simulink model "FOC_IM_1"  (R2021a)
settings: Solver=VariableStepAuto  StartTime=0.0  StopTime=10.0  RelTol=1e-3
values from neighbouring files (symbols this model uses):
  dataType = 'single'    [FOC_IM_1.m]
  inverter = mcb_SetInverterParameters('BoostXL-DRV8305')    [FOC_IM_1.m]
  PI_params = mcb.internal.SetControllerParameters(acim,inverter,PU_System,T_pwm,Ts,Ts_speed,Delays)    [FOC_IM_1.m]
  PU_System = mcb_SetPUSystem(acim,inverter)    [FOC_IM_1.m]
  target = mcb_SetProcessorDetails('F28379D',PWM_frequency)    [FOC_IM_1.m]
  Ts = T_pwm    (= 5e-05)    [FOC_IM_1.m]
  Ts_motor = T_pwm/2    (= 2.5e-05)    [FOC_IM_1.m]
  Ts_simulink = T_pwm/2    (= 2.5e-05)    [FOC_IM_1.m]
  Ts_speed = 30*Ts    (= 0.0015)    [FOC_IM_1.m]
undefined symbols (not defined in the file or in its folder): acim, IIR_filter_speed
libraries: mcbcontrolslib x21, simulink x8, c280xlib x3, mcbpositiondecoderlib x3, c2802xlib x2, autolibim x1, mcbplantlib x1, fuzblock x1
settings Model: Creator=ACER  LastModifiedBy=ACER

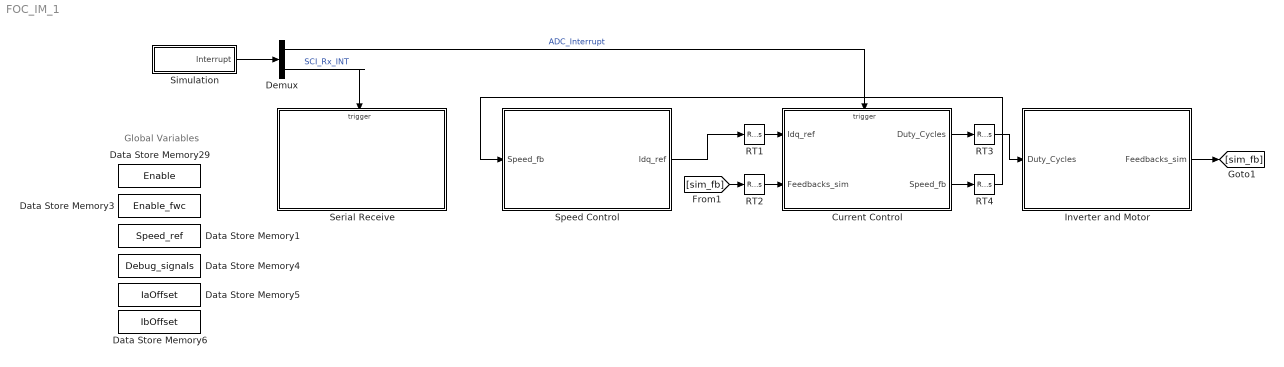
== system FOC_IM_1 ==
  note: Global Variables
  Current Control : Subsystem
      settings: RTWSystemCode=Nonreusable function
  Data Store Memory1 : DataStoreMemory  DataStoreName=Speed_ref  ReadBeforeWriteMsg=warning  WriteAfterWriteMsg=warning  WriteAfterReadMsg=warning  InitialValue=0.5  ShowAdditionalParam=off  OutDataTypeStr=dataType
  Data Store Memory29 : DataStoreMemory  DataStoreName=Enable  ReadBeforeWriteMsg=warning  WriteAfterWriteMsg=warning  WriteAfterReadMsg=warning  ShowAdditionalParam=off  OutDataTypeStr=boolean
  Data Store Memory3 : DataStoreMemory  DataStoreName=Enable_fwc  ReadBeforeWriteMsg=warning  WriteAfterWriteMsg=warning  WriteAfterReadMsg=warning  ShowAdditionalParam=off  OutDataTypeStr=boolean
  Data Store Memory4 : DataStoreMemory  DataStoreName=Debug_signals  ReadBeforeWriteMsg=warning  WriteAfterWriteMsg=warning  WriteAfterReadMsg=warning  InitialValue=5  ShowAdditionalParam=off  OutDataTypeStr=uint16
  Data Store Memory5 : DataStoreMemory  DataStoreName=IaOffset  InitialValue=inverter.CtSensAOffset  ShowAdditionalParam=off
  Data Store Memory6 : DataStoreMemory  DataStoreName=IbOffset  InitialValue=inverter.CtSensBOffset  ShowAdditionalParam=off
  Demux : Demux  Outputs=2
  Inverter and Motor : Subsystem
  RT1 : RateTransition  Deterministic=off
  RT2 : RateTransition  Deterministic=off
  RT3 : RateTransition  Deterministic=off
  RT4 : RateTransition  Deterministic=off  OutPortSampleTime=Ts_speed
  Serial Receive : Subsystem  SystemSampleTime=1e-3
  Simulation : Subsystem
  Speed Control : Subsystem  TreatAsAtomicUnit=on
      settings: RTWSystemCode=Nonreusable function
  wires:
  Demux/2 -> Serial Receive/Trigger  "SCI_Rx_INT"
  RT2/1 -> Current Control/2(Feedbacks_sim)
  Current Control/2(Speed_fb) -> RT4/1
  Current Control/1(Duty_Cycles) -> RT3/1
  RT3/1 -> Inverter and Motor/1(Duty_Cycles)
  [sim_fb] -> RT2/1
  Speed Control/1(Idq_ref) -> RT1/1
  Inverter and Motor/1(Feedbacks_sim) -> [sim_fb]
  RT4/1 -> Speed Control/1(Speed_fb)
  Demux/1 -> Current Control/Trigger  "ADC_Interrupt"
  RT1/1 -> Current Control/1(Idq_ref)
  Simulation/1(Interrupt) -> Demux/1

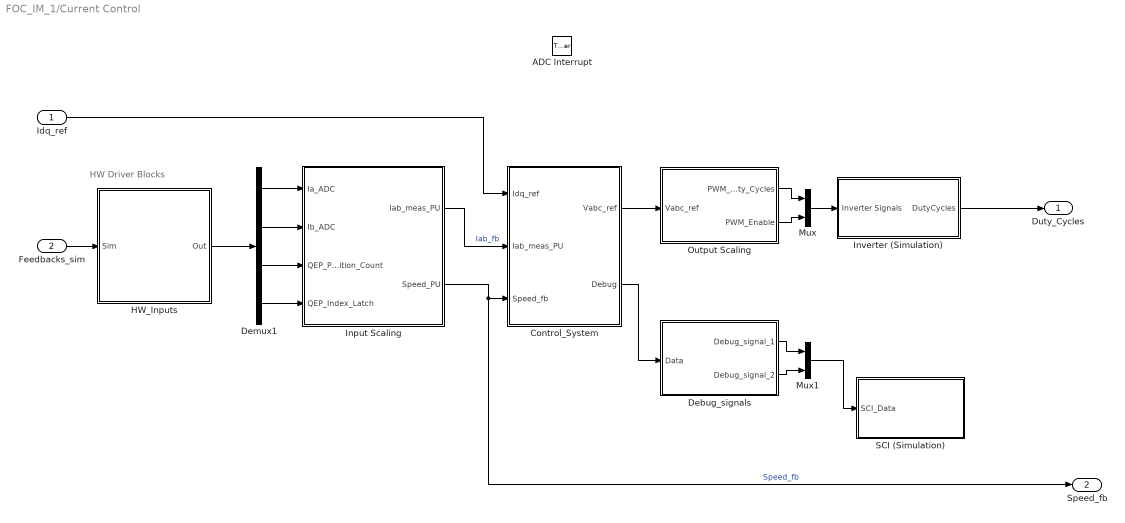
== system FOC_IM_1/Current Control ==
  note: HW Driver Blocks
  Idq_ref : Inport
  Feedbacks_sim : Inport  Port=2
  ADC Interrupt : TriggerPort  TriggerType=function-call  VariantControl=Variant
  Control_System : Subsystem
  Debug_signals : Subsystem
  Demux1 : Demux
  HW_Inputs : Subsystem  Variant=on  VariantControlMode=sim codegen switching
  Input Scaling : Subsystem
  Inverter (Simulation) : Subsystem
  Mux : Mux  Inputs=2
  Mux1 : Mux  Inputs=2
  Output Scaling : Subsystem
  SCI (Simulation) : Subsystem
  Duty_Cycles : Outport  InitialOutput=0  VectorParamsAs1DForOutWhenUnconnected=off
  Speed_fb : Outport  Port=2  InitialOutput=0  VectorParamsAs1DForOutWhenUnconnected=off
  wires:
  Input Scaling/2(Speed_PU) -> Control_System/3(Speed_fb), Speed_fb/1  "Speed_fb"
  Idq_ref/1 -> Control_System/1(Idq_ref)
  Control_System/1(Vabc_ref) -> Output Scaling/1(Vabc_ref)
  Input Scaling/1(Iab_meas_PU) -> Control_System/2(Iab_meas_PU)  "Iab_fb"
  Feedbacks_sim/1 -> HW_Inputs/1(Sim)
  Output Scaling/1(PWM_Duty_Cycles) -> Mux/1
  Output Scaling/2(PWM_Enable) -> Mux/2
  Mux1/1 -> SCI (Simulation)/1(SCI_Data)
  HW_Inputs/1(Out) -> Demux1/1
  Demux1/2 -> Input Scaling/2(Ib_ADC)
  Demux1/1 -> Input Scaling/1(Ia_ADC)
  Demux1/3 -> Input Scaling/3(QEP_Position_Count)
  Demux1/4 -> Input Scaling/4(QEP_Index_Latch)
  Control_System/2(Debug) -> Debug_signals/1(Data)
  Debug_signals/1(Debug_signal_1) -> Mux1/1
  Debug_signals/2(Debug_signal_2) -> Mux1/2
  Mux/1 -> Inverter (Simulation)/1(Inverter Signals)
  Inverter (Simulation)/1(DutyCycles) -> Duty_Cycles/1

== system FOC_IM_1/Inverter and Motor ==
  Duty_Cycles : Inport
  Simulation : Subsystem
  Feedbacks_sim : Outport  VectorParamsAs1DForOutWhenUnconnected=off
  wires:
  Duty_Cycles/1 -> Simulation/1(Duty_Cycles)
  Simulation/1(Feedbacks) -> Feedbacks_sim/1

== system FOC_IM_1/Serial Receive ==
  SCI_Rx_INT : TriggerPort  TriggerType=function-call  VariantControl=Variant
  Data Store Write : DataStoreWrite  DataStoreName=Enable  IndexOptions=Index vector (dialog)  Indices=1  OutputSizes=1
  Data Store Write1 : DataStoreWrite  DataStoreName=Debug_signals  IndexOptions=Index vector (dialog)  Indices=1  OutputSizes=1
  Data Store Write2 : DataStoreWrite  DataStoreName=Enable_fwc  IndexOptions=Index vector (dialog)  Indices=1  OutputSizes=1
  Data Store Write3 : DataStoreWrite  DataStoreName=Speed_ref  IndexOptions=Index vector (dialog)  Indices=1  OutputSizes=1
  Data_Conditioning_Rx : Subsystem  Variant=on
  Simulation : Subsystem
  unParse : Subsystem
  wires:
  Simulation/1(Out1) -> Data_Conditioning_Rx/1(In1)
  Data_Conditioning_Rx/1(Out1) -> Data Store Write3/1
  Data_Conditioning_Rx/2(Out2) -> unParse/1(Data)
  unParse/1(Enable_PWM) -> Data Store Write/1
  unParse/2(Enable_FWC) -> Data Store Write2/1
  unParse/3(Debug_signals) -> Data Store Write1/1

== system FOC_IM_1/Simulation ==
  ADCINT1 : simulink/Ports & Subsystems/Function-Call Generator  sample_time=Ts  numberOfIterations=1  DisallowWideOutput=off
  Mux : Mux  Inputs=2
  SCI_Rx_INT : simulink/Ports & Subsystems/Function-Call Generator  sample_time=0.1  numberOfIterations=1  DisallowWideOutput=off
  Interrupt : Outport
  wires:
  SCI_Rx_INT/1 -> Mux/2
  ADCINT1/1 -> Mux/1
  Mux/1 -> Interrupt/1

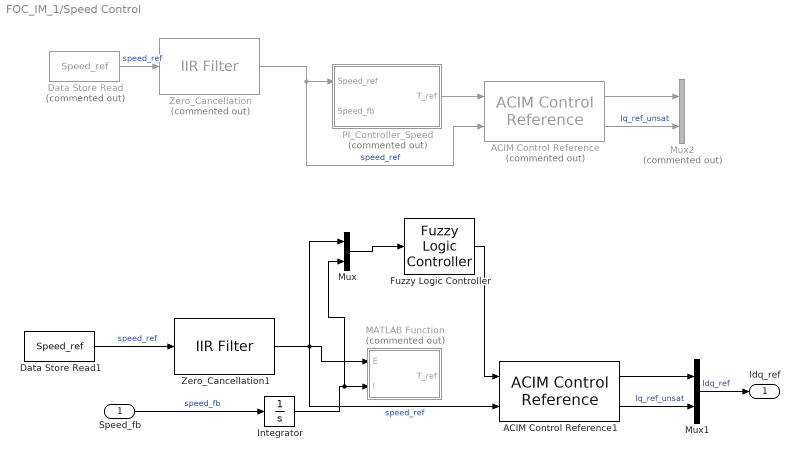
== system FOC_IM_1/Speed Control ==
  Speed_fb : Inport
  ACIM Control Reference : mcbcontrolslib/ACIM Control Reference  Commented=on  VariantControl=Surface PMSM  polePairs=acim.p  Llr=acim.Llr  Lm=acim.Lm  FluxRated=acim.FluxRated  N_rated=acim.N_rated  N_base=acim.N_base  I_sat=2*acim.I_rated  Units=Per-Unit (PU)  I_base=PU_System.I_base  T_base=0.75
      settings: SourceProductBaseCode=MT
  ACIM Control Reference1 : mcbcontrolslib/ACIM Control Reference  VariantControl=Surface PMSM  polePairs=acim.p  Llr=acim.Llr  Lm=acim.Lm  FluxRated=acim.FluxRated  N_rated=acim.N_rated  N_base=acim.N_base  I_sat=2*acim.I_rated  Units=Per-Unit (PU)  I_base=PU_System.I_base  T_base=0.42438
      settings: SourceProductBaseCode=MT
  Data Store Read : DataStoreRead  Commented=on  DataStoreName=Speed_ref  IndexOptions=Index vector (dialog)  Indices=1  OutputSizes=1
  Data Store Read1 : DataStoreRead  DataStoreName=Speed_ref  IndexOptions=Index vector (dialog)  Indices=1  OutputSizes=1
  Fuzzy Logic Controller : fuzblock/Fuzzy Logic  Controller  FIS=fuzzy_1  OutputSampleNumber=101  DataType=double  FuzzifiedInputs=off  RuleFiringStrengths=off  RuleOutputs=off  AggregatedOutputs=off  SimulateUsing=Interpreted execution  OutOfRangeInputValueMessage=warning  NoRuleFiredMessage=warning  EmptyOutputFuzzySetMessage=warning
  Integrator : Integrator  InitialCondition=Ts_speed
  MATLAB Function : MATLAB Function  Commented=on  TreatAsAtomicUnit=on
  Mux : Mux  Inputs=2
  Mux1 : Mux  Inputs=2
  Mux2 : Mux  Commented=on  Inputs=2
  PI_Controller_Speed : Subsystem  Commented=on
  Zero_Cancellation : mcbcontrolslib/IIR Filter  Commented=on  VariantControl=Low Pass Filter  VariantSelect=Low-pass  Filter_constant=IIR_filter_speed.coefficient * (Ts_speed / Ts)  advancedSettings=off  Ts=50e-6  cutOff_freq=1
      settings: SourceProductBaseCode=MT
  Zero_Cancellation1 : mcbcontrolslib/IIR Filter  VariantControl=Low Pass Filter  VariantSelect=Low-pass  Filter_constant=IIR_filter_speed.coefficient * (Ts_speed / Ts)  advancedSettings=off  Ts=50e-6  cutOff_freq=212.933
      settings: SourceProductBaseCode=MT
  Idq_ref : Outport  VectorParamsAs1DForOutWhenUnconnected=off
  wires:
  Data Store Read/1 -> Zero_Cancellation/1  "speed_ref"
  Zero_Cancellation/1 -> ACIM Control Reference/2, PI_Controller_Speed/1(Speed_ref)  "speed_ref"
  PI_Controller_Speed/1(T_ref) -> ACIM Control Reference/1
  ACIM Control Reference/1 -> Mux2/1
  ACIM Control Reference/2 -> Mux2/2  "Iq_ref_unsat"
  ACIM Control Reference1/2 -> Mux1/2  "Iq_ref_unsat"
  ACIM Control Reference1/1 -> Mux1/1
  Data Store Read1/1 -> Zero_Cancellation1/1  "speed_ref"
  Zero_Cancellation1/1 -> Mux/1, ACIM Control Reference1/2, MATLAB Function/1(E)  "speed_ref"
  Integrator/1 -> Mux/2, MATLAB Function/2(I)
  Speed_fb/1 -> Integrator/1  "speed_fb"
  Mux1/1 -> Idq_ref/1  "Idq_ref"
  Mux/1 -> Fuzzy Logic Controller/1
  Fuzzy Logic Controller/1 -> ACIM Control Reference1/1

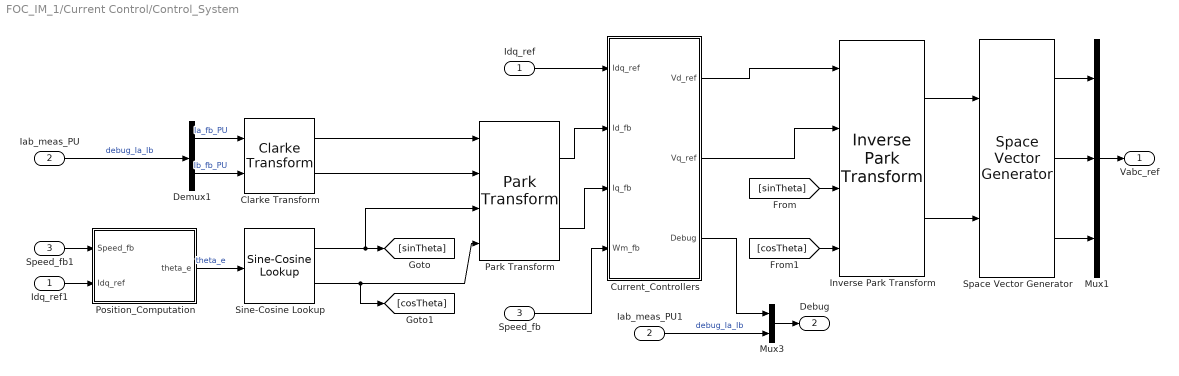
== system FOC_IM_1/Current Control/Control_System ==
  Idq_ref : Inport
  Iab_meas_PU : Inport  Port=2
  Speed_fb : Inport  Port=3
  Clarke Transform : mcbcontrolslib/Clarke Transform  VariantControl=Variant2
  Current_Controllers : Subsystem
  Demux1 : Demux  Outputs=2
  Iab_meas_PU1 : InportShadow  Port=2
  Idq_ref1 : InportShadow
  Inverse Park Transform : mcbcontrolslib/Inverse Park Transform  AxisAlignment=D-axis
  Mux1 : Mux  Inputs=3
  Mux3 : Mux  Inputs=2
  Park Transform : mcbcontrolslib/Park Transform  AxisAlignment=D-axis
      settings: SourceProductBaseCode=MT
  Position_Computation : Subsystem
  Sine-Cosine Lookup : mcbcontrolslib/Sine-Cosine Lookup  AngleInput=Per-unit  N_points=1024
      settings: SourceProductBaseCode=MT
  Space Vector Generator : mcbcontrolslib/Space Vector Generator
      settings: SourceProductBaseCode=MT
  Speed_fb1 : InportShadow  Port=3
  Vabc_ref : Outport  VectorParamsAs1DForOutWhenUnconnected=off
  Debug : Outport  Port=2  VectorParamsAs1DForOutWhenUnconnected=off
  wires:
  Park Transform/1 -> Current_Controllers/2(Id_fb)
  Inverse Park Transform/1 -> Space Vector Generator/1
  Inverse Park Transform/2 -> Space Vector Generator/2
  Sine-Cosine Lookup/1 -> Park Transform/3, [sinTheta]
  Sine-Cosine Lookup/2 -> Park Transform/4, [cosTheta]
  [cosTheta] -> Inverse Park Transform/4
  [sinTheta] -> Inverse Park Transform/3
  Clarke Transform/2 -> Park Transform/2
  Clarke Transform/1 -> Park Transform/1
  Idq_ref/1 -> Current_Controllers/1(Idq_ref)
  Space Vector Generator/1 -> Mux1/1
  Space Vector Generator/2 -> Mux1/2
  Current_Controllers/1(Vd_ref) -> Inverse Park Transform/1
  Current_Controllers/2(Vq_ref) -> Inverse Park Transform/2
  Space Vector Generator/3 -> Mux1/3
  Mux1/1 -> Vabc_ref/1
  Demux1/1 -> Clarke Transform/1  "Ia_fb_PU"
  Demux1/2 -> Clarke Transform/2  "Ib_fb_PU"
  Iab_meas_PU/1 -> Demux1/1  "debug_Ia_Ib"
  Iab_meas_PU1/1 -> Mux3/2  "debug_Ia_Ib"
  Current_Controllers/3(Debug) -> Mux3/1
  Mux3/1 -> Debug/1
  Park Transform/2 -> Current_Controllers/3(Iq_fb)
  Speed_fb/1 -> Current_Controllers/4(Wm_fb)
  Position_Computation/1(theta_e) -> Sine-Cosine Lookup/1  "theta_e"
  Speed_fb1/1 -> Position_Computation/1(Speed_fb)
  Idq_ref1/1 -> Position_Computation/2(Idq_ref)

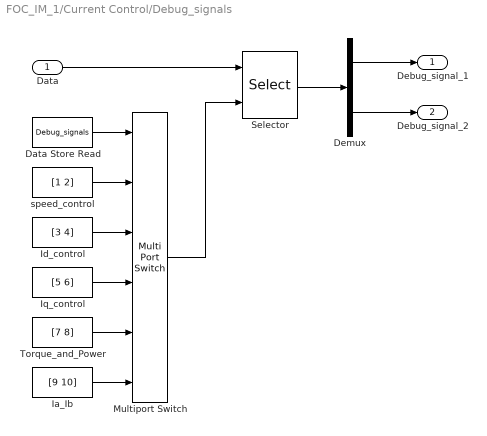
== system FOC_IM_1/Current Control/Debug_signals ==
  Data : Inport
  Data Store Read : DataStoreRead  DataStoreName=Debug_signals  IndexOptions=Index vector (dialog)  Indices=1  OutputSizes=1
  Demux : Demux  Outputs=2
  Ia_Ib : Constant  Value=[9 10]  OutDataTypeStr=uint16  SampleTime=-1
  Id_control : Constant  Value=[3 4]  OutDataTypeStr=uint16  SampleTime=-1
  Iq_control : Constant  Value=[5 6]  OutDataTypeStr=uint16  SampleTime=-1
  Multiport Switch : MultiPortSwitch  Inputs=5  DiagnosticForDefault=Warning  OutDataTypeStr=uint16  RndMeth=Simplest
  Selector : Selector  InputPortWidth=10  IndexOptions=Index vector (port)  Indices=[1 3]  OutputSizes=1
  Torque_and_Power : Constant  Value=[7 8]  OutDataTypeStr=uint16  SampleTime=-1
  speed_control : Constant  Value=[1 2]  OutDataTypeStr=uint16  SampleTime=-1
  Debug_signal_1 : Outport
  Debug_signal_2 : Outport  Port=2
  wires:
  Data/1 -> Selector/1
  Demux/2 -> Debug_signal_2/1
  speed_control/1 -> Multiport Switch/2
  Selector/1 -> Demux/1
  Demux/1 -> Debug_signal_1/1
  Id_control/1 -> Multiport Switch/3
  Iq_control/1 -> Multiport Switch/4
  Torque_and_Power/1 -> Multiport Switch/5
  Ia_Ib/1 -> Multiport Switch/6
  Multiport Switch/1 -> Selector/2
  Data Store Read/1 -> Multiport Switch/1

== system FOC_IM_1/Current Control/HW_Inputs ==
  Sim : Inport
  Sensor Driver Blocks (codegen) : Subsystem  VariantControl=(codegen)
  Sensor Driver Blocks (sim) : Subsystem  VariantControl=(sim)
  Out : Outport

== system FOC_IM_1/Current Control/Input Scaling ==
  note: Current Measurements
  note: Position & Speed Measurements
  Ia_ADC : Inport
  Ib_ADC : Inport  Port=2
  QEP_Position_Count : Inport  Port=3
  QEP_Index_Latch : Inport  Port=4
  Calculate Phase Currents : Subsystem
  Calculate position and speed : Subsystem
  Demux : Demux  Outputs=2
  Terminator : Terminator
  Iab_meas_PU : Outport
  Speed_PU : Outport  Port=2
  wires:
  Calculate Phase Currents/1(Iab_meas_PU) -> Iab_meas_PU/1  "Iab_fb_PU"
  Ia_ADC/1 -> Calculate Phase Currents/1(Ia_ADC)
  Ib_ADC/1 -> Calculate Phase Currents/2(Ib_ADC)
  QEP_Index_Latch/1 -> Calculate position and speed/2(QEP_Index_Latch)
  QEP_Position_Count/1 -> Calculate position and speed/1(QEP_Position_Count)
  Demux/1 -> Terminator/1
  Demux/2 -> Speed_PU/1  "speed_fb_sensors"
  Calculate position and speed/1(Pos/Speed) -> Demux/1

== system FOC_IM_1/Current Control/Inverter (Simulation) ==
  Inverter Signals : Inport
  Data Type Duplicate : DataTypeDuplicate
  Demux : Demux
  Mux : Mux  Inputs=3
  Mux2 : Mux  Inputs=3
  Switch1 : Switch  Threshold=0.5  RndMeth=Simplest
  stop : Constant  Value=0  OutDataTypeStr=Inherit: Inherit via back propagation
  DutyCycles : Outport  VectorParamsAs1DForOutWhenUnconnected=off
  wires:
  stop/1 -> Data Type Duplicate/2, Mux2/1, Mux2/3, Mux2/2
  Mux2/1 -> Switch1/3
  Switch1/1 -> DutyCycles/1
  Inverter Signals/1 -> Demux/1
  Demux/4 -> Switch1/2  "PWM Enable"
  Mux/1 -> Data Type Duplicate/1, Switch1/1  "PWM Duty Cycles"
  Demux/1 -> Mux/1
  Demux/2 -> Mux/2
  Demux/3 -> Mux/3

== system FOC_IM_1/Current Control/Output Scaling ==
  Vabc_ref : Inport
  Constant : Constant  Value=0.5  OutDataTypeStr=dataType  SampleTime=-1
  Data Type Conversion : DataTypeConversion  OutDataTypeStr=dataType
  Enable : DataStoreRead  DataStoreName=Enable  IndexOptions=Index vector (dialog)  Indices=1  OutputSizes=1
  One_by_Two : Gain  Gain=0.5  RndMeth=Simplest  OutDataTypeStr=Inherit: Same as input
  Sum : Sum  Inputs=|++
  PWM_Duty_Cycles : Outport
  PWM_Enable : Outport  Port=2
  wires:
  Constant/1 -> Sum/2
  Vabc_ref/1 -> One_by_Two/1
  Sum/1 -> PWM_Duty_Cycles/1  "PWM_Duty_Cycles"
  Enable/1 -> Data Type Conversion/1  "PWM_En"
  One_by_Two/1 -> Sum/1
  Data Type Conversion/1 -> PWM_Enable/1

== system FOC_IM_1/Current Control/SCI (Simulation) ==
  SCI_Data : Inport
  Demux : Demux  Outputs=2
  Terminator1 : Terminator
  Terminator2 : Terminator
  wires:
  SCI_Data/1 -> Demux/1
  Demux/1 -> Terminator1/1
  Demux/2 -> Terminator2/1

== system FOC_IM_1/Inverter and Motor/Simulation ==
  Duty_Cycles : Inport
  Load_Profile (Torque) : Subsystem
  Motor and Inverter : Subsystem  VariantControl=(get_param([bdroot '/InverterSelected'], 'Value') == '0')
  RT1 : RateTransition  Deterministic=off  OutPortSampleTime=Ts_simulink
  RT3 : RateTransition  Deterministic=off  OutPortSampleTime=Ts_simulink
  Sensor_Measurements : Subsystem
  Feedbacks : Outport  VectorParamsAs1DForOutWhenUnconnected=off
  wires:
  Sensor_Measurements/1(Sim_fb) -> Feedbacks/1
  Load_Profile (Torque)/1(Load_Trq) -> Motor and Inverter/2(Load)
  Motor and Inverter/1(Iabc) -> RT1/1  "Iabc"
  Duty_Cycles/1 -> Motor and Inverter/1(Vabc_In_PU)
  RT3/1 -> Sensor_Measurements/2(pos)
  Motor and Inverter/2(Theta) -> RT3/1
  RT1/1 -> Sensor_Measurements/1(PhaseCurr)

== system FOC_IM_1/Serial Receive/Data_Conditioning_Rx ==
  In1 : Inport
  Data_Type_Float : Subsystem  VariantControl=isequal(dataType, 'single')
  Out1 : Outport
  Out2 : Outport  Port=2

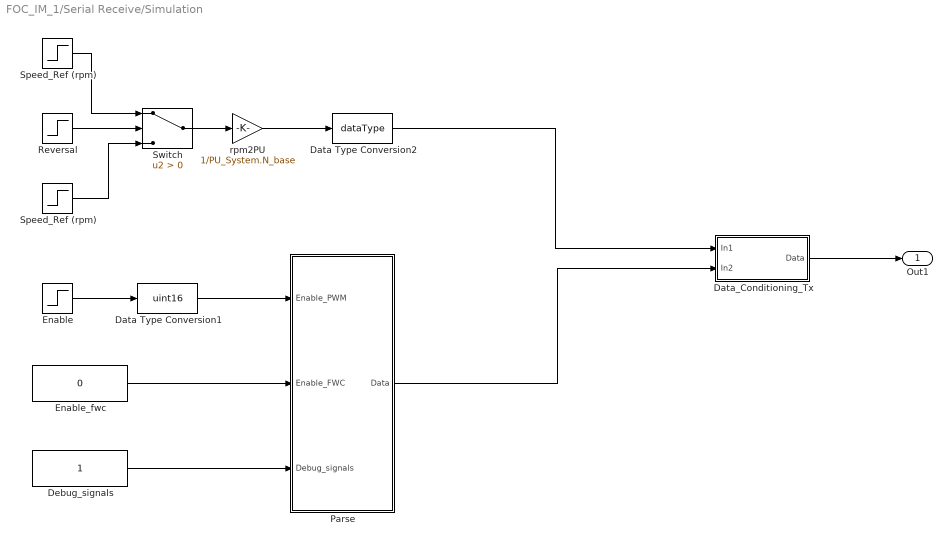
== system FOC_IM_1/Serial Receive/Simulation ==
  Data Type Conversion1 : DataTypeConversion  OutDataTypeStr=uint16  RndMeth=Simplest
  Data Type Conversion2 : DataTypeConversion  OutDataTypeStr=dataType  RndMeth=Simplest
  Data_Conditioning_Tx : Subsystem  Variant=on
  Debug_signals : Constant  OutDataTypeStr=uint16  SampleTime=-1
  Enable : Step  Time=0.1
  Enable_fwc : Constant  Value=0  OutDataTypeStr=uint16  SampleTime=-1
  Parse : Subsystem
  Reversal : Step  Time=9
  Speed_Ref (rpm) : Step  Time=6  Before=0.5*acim.N_rated  After=0.8*acim.N_rated
  Speed_Ref (rpm) : Step  Time=4  Before=0.8*acim.N_rated  After=-0.8*acim.N_rated
  Switch : Switch  Criteria=u2 > Threshold
  rpm2PU : Gain  Gain=1/PU_System.N_base  RndMeth=Simplest  OutDataTypeStr=Inherit: Same as input
  Out1 : Outport
  wires:
  Data_Conditioning_Tx/1(Data) -> Out1/1
  Speed_Ref (rpm)/1 -> Switch/3
  rpm2PU/1 -> Data Type Conversion2/1
  Data Type Conversion1/1 -> Parse/1(Enable_PWM)
  Enable_fwc/1 -> Parse/2(Enable_FWC)
  Debug_signals/1 -> Parse/3(Debug_signals)
  Parse/1(Data) -> Data_Conditioning_Tx/2(In2)
  Speed_Ref (rpm)/1 -> Switch/1
  Reversal/1 -> Switch/2
  Switch/1 -> rpm2PU/1
  Data Type Conversion2/1 -> Data_Conditioning_Tx/1(In1)
  Enable/1 -> Data Type Conversion1/1

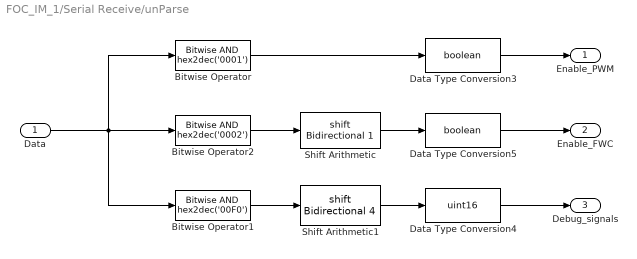
== system FOC_IM_1/Serial Receive/unParse ==
  Data : Inport
  Bitwise Operator : simulink/Logic and Bit Operations/Bitwise Operator  logicop=AND  UseBitMask=on  BitMask=hex2dec('0001')  BitMaskRealWorld=Stored Integer
  Bitwise Operator1 : simulink/Logic and Bit Operations/Bitwise Operator  logicop=AND  UseBitMask=on  BitMask=hex2dec('00F0')  BitMaskRealWorld=Stored Integer
  Bitwise Operator2 : simulink/Logic and Bit Operations/Bitwise Operator  logicop=AND  UseBitMask=on  BitMask=hex2dec('0002')  BitMaskRealWorld=Stored Integer
  Data Type Conversion3 : DataTypeConversion  OutDataTypeStr=boolean  RndMeth=Simplest
  Data Type Conversion4 : DataTypeConversion  OutDataTypeStr=uint16  RndMeth=Simplest
  Data Type Conversion5 : DataTypeConversion  OutDataTypeStr=boolean  RndMeth=Simplest
  Shift Arithmetic : ArithShift  BitShiftNumber=1
  Shift Arithmetic1 : ArithShift  BitShiftNumber=4
  Enable_PWM : Outport
  Enable_FWC : Outport  Port=2
  Debug_signals : Outport  Port=3
  wires:
  Bitwise Operator2/1 -> Shift Arithmetic/1
  Bitwise Operator1/1 -> Shift Arithmetic1/1
  Data/1 -> Bitwise Operator/1, Bitwise Operator2/1, Bitwise Operator1/1
  Bitwise Operator/1 -> Data Type Conversion3/1
  Data Type Conversion4/1 -> Debug_signals/1
  Shift Arithmetic1/1 -> Data Type Conversion4/1
  Data Type Conversion3/1 -> Enable_PWM/1
  Shift Arithmetic/1 -> Data Type Conversion5/1
  Data Type Conversion5/1 -> Enable_FWC/1

== system FOC_IM_1/Speed Control/PI_Controller_Speed ==
  Speed_ref : Inport
  Speed_fb : Inport  Port=2
  Data Store Read2 : DataStoreRead  DataStoreName=Enable  IndexOptions=Index vector (dialog)  Indices=1  OutputSizes=1
  Discrete PI Controller with anti-windup & reset : mcbcontrolslib/Discrete PI Controller  with anti-windup & reset  UpperSaturationLimit=1  LowerSaturationLimit=-1
      settings: SourceProductBaseCode=MT
  Ki1 : Constant  Value=PI_params.Ki_speed*Ts_speed  OutDataTypeStr=dataType  SampleTime=-1
  Ki2 : Constant  Value=0  OutDataTypeStr=dataType  SampleTime=-1
  Kp1 : Constant  Value=PI_params.Kp_speed  OutDataTypeStr=dataType  SampleTime=-1
  Logical Operator : Logic  Operator=NOT  IconShape=distinctive  AllPortsSameDT=off  OutDataTypeStr=boolean
  Sum : Sum  Inputs=|+-
  T_ref : Outport  VectorParamsAs1DForOutWhenUnconnected=off
  wires:
  Discrete PI Controller with anti-windup & reset/1 -> T_ref/1
  Ki1/1 -> Discrete PI Controller with anti-windup & reset/3
  Kp1/1 -> Discrete PI Controller with anti-windup & reset/2
  Speed_fb/1 -> Sum/2
  Speed_ref/1 -> Sum/1
  Sum/1 -> Discrete PI Controller with anti-windup & reset/1
  Logical Operator/1 -> Discrete PI Controller with anti-windup & reset/4
  Data Store Read2/1 -> Logical Operator/1
  Ki2/1 -> Discrete PI Controller with anti-windup & reset/5

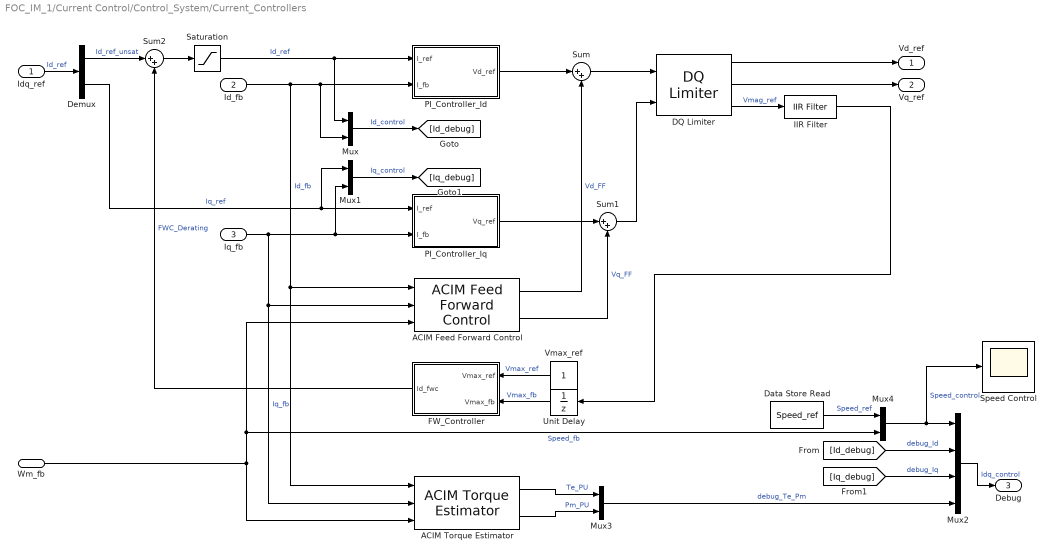
== system FOC_IM_1/Current Control/Control_System/Current_Controllers ==
  Idq_ref : Inport
  Id_fb : Inport  Port=2
  Iq_fb : Inport  Port=3
  Wm_fb : Inport  Port=4
  ACIM Feed Forward Control : mcbcontrolslib/ACIM Feed Forward Control  polePairs=acim.p  Lls=acim.Lls  Llr=acim.Llr  Lm=acim.Lm  FluxRated=acim.FluxRated  V_dc=0.5*PU_System.V_base  Units=Per-Unit (PU)  V_base=PU_System.V_base  I_base=PU_System.I_base  N_base=PU_System.N_base
      settings: SourceProductBaseCode=MT
  ACIM Torque Estimator : mcbcontrolslib/ACIM Torque Estimator  polePairs=acim.p  Lls=acim.Lls  Llr=acim.Llr  Lm=acim.Lm  FluxRated=acim.FluxRated  Units=Per-Unit (PU)  V_base=PU_System.V_base  I_base=PU_System.I_base  N_base=PU_System.N_base  T_base=0.42438  P_base=120.625
      settings: SourceProductBaseCode=MT
  DQ Limiter : mcbcontrolslib/DQ Limiter  Vmax=0.9
      settings: SourceProductBaseCode=MT
  Data Store Read : DataStoreRead  DataStoreName=Speed_ref  IndexOptions=Index vector (dialog)  Indices=1  OutputSizes=1
  Demux : Demux  Outputs=2
  FW_Controller : Subsystem
  IIR Filter : mcbcontrolslib/IIR Filter  VariantControl=Low Pass Filter  VariantSelect=Low-pass  Filter_constant=0.01  advancedSettings=off  Ts=50e-6  cutOff_freq=32.1525
      settings: SourceProductBaseCode=MT
  Mux{,1,3..4} (4 alike) : Mux  Inputs=2
  Mux2 : Mux
  PI_Controller_Id : Subsystem
  PI_Controller_Iq : Subsystem
  Saturation : Saturate  LowerLimit=0.05
  Speed Control : Scope
  Sum : Sum  Inputs=|++
  Sum1 : Sum  Inputs=|++
  Sum2 : Sum  Inputs=|++
  Unit Delay : UnitDelay  SampleTime=-1  HasFrameUpgradeWarning=on
  Vmax_ref : Constant  OutDataTypeStr=dataType  SampleTime=-1
  Vd_ref : Outport  VectorParamsAs1DForOutWhenUnconnected=off
  Vq_ref : Outport  Port=2  VectorParamsAs1DForOutWhenUnconnected=off
  Debug : Outport  Port=3  VectorParamsAs1DForOutWhenUnconnected=off
  wires:
  Mux/1 -> [Id_debug]  "Id_control"
  Id_fb/1 -> ACIM Torque Estimator/1, ACIM Feed Forward Control/1, Mux/2, PI_Controller_Id/2(I_fb)  "Id_fb"
  Mux1/1 -> [Iq_debug]  "Iq_control"
  DQ Limiter/1 -> Vd_ref/1
  DQ Limiter/2 -> Vq_ref/1
  PI_Controller_Id/1(Vd_ref) -> Sum/1
  ACIM Torque Estimator/1 -> Mux3/1  "Te_PU"
  Iq_fb/1 -> ACIM Torque Estimator/2, ACIM Feed Forward Control/2, PI_Controller_Iq/2(I_fb), Mux1/2  "Iq_fb"
  PI_Controller_Iq/1(Vq_ref) -> Sum1/1
  Sum1/1 -> DQ Limiter/2
  Demux/2 -> Mux1/1, PI_Controller_Iq/1(I_ref)  "Iq_ref"
  Idq_ref/1 -> Demux/1  "Id_ref"
  Mux2/1 -> Debug/1  "Idq_control"
  [Id_debug] -> Mux2/2  "debug_Id"
  [Iq_debug] -> Mux2/3  "debug_Iq"
  ACIM Torque Estimator/2 -> Mux3/2  "Pm_PU"
  Mux3/1 -> Mux2/4  "debug_Te_Pm"
  Mux4/1 -> Speed Control/1, Mux2/1  "Speed_control"
  Wm_fb/1 -> ACIM Feed Forward Control/3, Mux4/2, ACIM Torque Estimator/3  "Speed_fb"
  Data Store Read/1 -> Mux4/1  "Speed_ref"
  Sum2/1 -> Saturation/1
  Sum/1 -> DQ Limiter/1
  IIR Filter/1 -> Unit Delay/1
  ACIM Feed Forward Control/1 -> Sum/2  "Vd_FF"
  ACIM Feed Forward Control/2 -> Sum1/2  "Vq_FF"
  Unit Delay/1 -> FW_Controller/2(Vmax_fb)  "Vmax_fb"
  Vmax_ref/1 -> FW_Controller/1(Vmax_ref)  "Vmax_ref"
  Demux/1 -> Sum2/1  "Id_ref_unsat"
  FW_Controller/1(Id_fwc) -> Sum2/2  "FWC_Derating"
  Saturation/1 -> PI_Controller_Id/1(I_ref), Mux/1  "Id_ref"
  DQ Limiter/3 -> IIR Filter/1  "Vmag_ref"

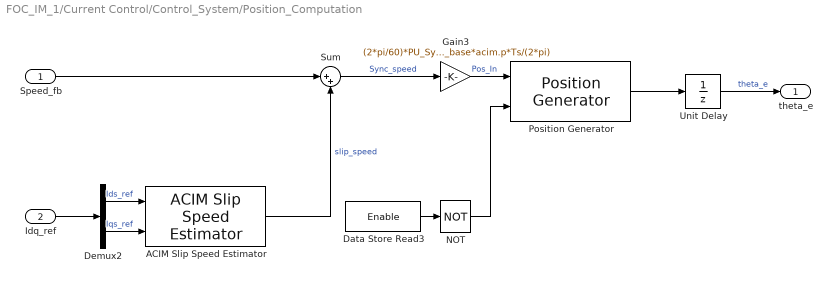
== system FOC_IM_1/Current Control/Control_System/Position_Computation ==
  Speed_fb : Inport
  Idq_ref : Inport  Port=2
  ACIM Slip Speed Estimator : mcbcontrolslib/ACIM Slip Speed Estimator  polePairs=acim.p  Rr=acim.Rr  Llr=acim.Llr  Lm=acim.Lm  N_sat=acim.N_base - acim.N_rated  Units=Per-Unit (PU)  N_base=acim.N_base
      settings: SourceProductBaseCode=MT
  Data Store Read3 : DataStoreRead  DataStoreName=Enable  IndexOptions=Index vector (dialog)  Indices=1  OutputSizes=1
  Demux2 : Demux  Outputs=2
  Gain3 : Gain  Gain=(2*pi/60)*PU_System.N_base*acim.p*Ts/(2*pi)  RndMeth=Simplest  OutDataTypeStr=Inherit: Same as input
  NOT : Logic  Operator=NOT  IconShape=distinctive  AllPortsSameDT=off  OutDataTypeStr=boolean
  Position Generator : mcbcontrolslib/Position Generator  AngleOutput=Per-unit  ThetaSource=External  ThetaInput=5e-4  DataType=double  ExternalReset=active high resets to zero  Offset=0
      settings: SourceProductBaseCode=MT
  Sum : Sum  Inputs=|++
  Unit Delay : UnitDelay  SampleTime=-1  HasFrameUpgradeWarning=on
  theta_e : Outport
  wires:
  Position Generator/1 -> Unit Delay/1
  Sum/1 -> Gain3/1  "Sync_speed"
  Demux2/1 -> ACIM Slip Speed Estimator/1  "Ids_ref"
  Data Store Read3/1 -> NOT/1
  ACIM Slip Speed Estimator/1 -> Sum/2  "slip_speed"
  Gain3/1 -> Position Generator/1  "Pos_In"
  NOT/1 -> Position Generator/2
  Demux2/2 -> ACIM Slip Speed Estimator/2  "Iqs_ref"
  Idq_ref/1 -> Demux2/1
  Speed_fb/1 -> Sum/1
  Unit Delay/1 -> theta_e/1  "theta_e"

== system FOC_IM_1/Current Control/HW_Inputs/Sensor Driver Blocks (codegen) ==
  Sim : Inport
  ADC_B_IN2 : c2802xlib/ADC  blkParamProc=C2000_Type4  ADCModule=B  samplingMode=Single sample mode  ADCResolution=12-bit (Single-ended input)  useSOC1=SOC0  useSOC2=SOC0_SOC1  SOCAcquisitionWindow=15  SOCTriggerSource=ePWM1_ADCSOCA  SOCInterruptTrigger=No ADCINT  Ts=-1  dType=uint16  postInterrupt=on  interruptSel=ADCINT1  ADCINTContinuous=on  endma=off  chdma=1  conv1=ADCINA0  conv2=ADCINA0 and ADCINB0  conv1_Type4=ADCIN2  conv2_Type4=ADCIN0 and ADCIN1
  ADC_C_IN2 : c2802xlib/ADC  blkParamProc=C2000_Type4  ADCModule=C  samplingMode=Single sample mode  ADCResolution=12-bit (Single-ended input)  useSOC1=SOC0  useSOC2=SOC0_SOC1  SOCAcquisitionWindow=15  SOCTriggerSource=ePWM1_ADCSOCA  SOCInterruptTrigger=No ADCINT  Ts=-1  dType=uint16  postInterrupt=off  interruptSel=ADCINT1  ADCINTContinuous=on  endma=off  chdma=1  conv1=ADCINA0  conv2=ADCINA0 and ADCINB0  conv1_Type4=ADCIN2  conv2_Type4=ADCIN0 and ADCIN1
  Mux1 : Mux
  Optional_Read_SPI : Subsystem  Commented=on
  Terminator : Terminator
  eQEP : c280xlib/eQEP  useModule=eQEP1  pcInputmode=Quadrature-count  externalClockrate=2x resolution: Count the rising/falling edge  swapPolarityselection=Counterclockwise  qdfOutputport=off  qapPolarityselection=on  qbpPolarityselection=on  qipPolarityselection=on  qspPolarityselection=off  igatePolarityselection=off  sampleTime=-1  pcOutputport=on  pcMaximumvalue=2^16-1  indexInitializationcheck=off  indexInitializationevent=Rising edge  strobeInitializationcheck=off  strobeInitializationevent=Rising edge  softwareInitializationcheck=off  softwareInitializationsource=Set to init value at start up  softwareInitializationmode=on  pcInitialvalue=2147483648  pcResetmode=Reset on the first index event  ieloutputport=on  indexEventlatch=Falling edge  seloutputport=off  strobeEventlatch=Rising edge  pcefOutputport=off  enableEqepcapture=off  qctmrOutputport=off  qcprdOutputport=off  captureTimerprescaler=128  upEventprescaler=128  overflowErrorflag=off  directionErrorflag=off  captureTimerposition=On position counter read  unitTimerperiod=100000000  captureTimerlatch=off  capturePeriodlatch=off  positionCounterlatch=off  soenPolarityselection=off  spselPolarityselection=Index pin is used for sync output  compareValuesource=Specify via dialog  shadowMode=Load on QPOSCNT=0  compareValue=4294967295  syncOutputwidth=1  polaritySyncoutput=Active high  watchdogEnable=off  watchdogTimer=65535  outport1Datatype=auto  outport2Datatype=auto  outport3Datatype=auto  outport4Datatype=auto  outport5Datatype=auto  outport6Datatype=auto  outport7Datatype=auto  outport8Datatype=auto  outport9Datatype=auto  outport10Datatype=auto  outport11Datatype=auto  outport12Datatype=auto  eqepinterrupt_pce=off  eqepinterrupt_qpe=off  eqepinterrupt_qdc=off  eqepinterrupt_wto=off  eqepinterrupt_pcu=off  eqepinterrupt_pco=off  eqepinterrupt_pcr=off  eqepinterrupt_pcm=off  eqepinterrupt_sel=off  eqepinterrupt_iel=off  eqepinterrupt_uto=off  pheOutputport=off  watchdogOutputport=off  outport13Datatype=auto  outport14Datatype=auto
      settings: SourceProductBaseCode=TIC2000
  Out : Outport
  wires:
  ADC_C_IN2/1 -> Mux1/1
  Mux1/1 -> Out/1
  ADC_B_IN2/1 -> Mux1/2
  Sim/1 -> Terminator/1
  eQEP/1 -> Mux1/3
  eQEP/2 -> Mux1/4

== system FOC_IM_1/Current Control/HW_Inputs/Sensor Driver Blocks (sim) ==
  Sim : Inport
  Out : Outport
  wires:
  Sim/1 -> Out/1

== system FOC_IM_1/Current Control/Input Scaling/Calculate Phase Currents ==
  Ia_ADC : Inport
  Ib_ADC : Inport  Port=2
  Add : Sum  Inputs=-+
  Data Store Read1 : DataStoreRead  DataStoreName=IaOffset  IndexOptions=Index vector (dialog)  Indices=1  OutputSizes=1
  Data Store Read2 : DataStoreRead  DataStoreName=IbOffset  IndexOptions=Index vector (dialog)  Indices=1  OutputSizes=1
  Data Type Conversion : DataTypeConversion  OutDataTypeStr=int32  ConvertRealWorld=Stored Integer (SI)  RndMeth=Simplest
  Data_Type : Subsystem  Variant=on
  Inverting / Non-inverting Current measurement amplifieer : Gain  Gain=inverter.invertingAmp  RndMeth=Simplest  OutDataTypeStr=Inherit: Same as input
  Mux : Mux  Inputs=2
  Mux1 : Mux  Inputs=2
  Iab_meas_PU : Outport  VectorParamsAs1DForOutWhenUnconnected=off
  wires:
  Data Type Conversion/1 -> Add/2
  Add/1 -> Data_Type/1(In1)
  Ia_ADC/1 -> Mux/1
  Ib_ADC/1 -> Mux/2
  Mux/1 -> Data Type Conversion/1
  Mux1/1 -> Add/1
  Data Store Read1/1 -> Mux1/1
  Data Store Read2/1 -> Mux1/2
  Data_Type/1(Out1) -> Inverting / Non-inverting Current measurement amplifieer/1
  Inverting / Non-inverting Current measurement amplifieer/1 -> Iab_meas_PU/1

== system FOC_IM_1/Current Control/Input Scaling/Calculate position and speed ==
  QEP_Position_Count : Inport
  QEP_Index_Latch : Inport  Port=2
  IIR Filter : mcbcontrolslib/IIR Filter  VariantControl=Low Pass Filter  VariantSelect=Low-pass  Filter_constant=IIR_filter_speed.coefficient  advancedSettings=off  Ts=50e-6  cutOff_freq=6.6667
      settings: SourceProductBaseCode=MT
  IndexOffset : Constant  Value=acim.PositionOffset  OutDataTypeStr=dataType  SampleTime=-1
  Mechanical to Electrical Position : mcbpositiondecoderlib/Mechanical to Electrical Position  NrPP=acim.p  selectedRange=Per unit  MechOfstInputType=Input port  mechOffsetIn=0  maxAngleIn=1  InputDataType=dataType  VariantSelect=fixed-point
      settings: SourceProductBaseCode=MT
  Mux : Mux  Inputs=2
  Quadrature Decoder : mcbpositiondecoderlib/Quadrature Decoder  EncoderSlitsPerRevolution=acim.QEPSlits  EncoderCountsPerSlit=4  CounterSize=16 bits  ExternalIndexCount=on  PositionUnit=Per unit  PositionDataType=dataType
      settings: SourceProductBaseCode=MT
  Speed Measurement : mcbpositiondecoderlib/Speed Measurement  PositionUnit=Per unit  SpeedCalculationMode=Maximum application speed  SampleTimeAsync=Ts  MaximumApplicationSpeed=2*PU_System.N_base  SpeedResolution=5e-6  DelayLength=199  MaximumMeasurableSpeed=3000  MeasurableSpeedResolution=1.397e-06  SpeedUnit=Per unit based on dialog  PerUnitSpeed=PU_System.N_base  SpeedDataType=dataType
      settings: SourceProductBaseCode=MT
  Pos/Speed : Outport  VectorParamsAs1DForOutWhenUnconnected=off
  wires:
  QEP_Index_Latch/1 -> Quadrature Decoder/2
  QEP_Position_Count/1 -> Quadrature Decoder/1
  Speed Measurement/1 -> IIR Filter/1
  Mechanical to Electrical Position/1 -> Mux/1
  Quadrature Decoder/1 -> Mechanical to Electrical Position/1, Speed Measurement/1
  Mux/1 -> Pos/Speed/1
  IIR Filter/1 -> Mux/2
  IndexOffset/1 -> Mechanical to Electrical Position/2

== system FOC_IM_1/Inverter and Motor/Simulation/Load_Profile (Torque) ==
  Data Type Conversion : DataTypeConversion  OutDataTypeStr=single
  IIR Filter : mcbcontrolslib/IIR Filter  VariantControl=Low Pass Filter  VariantSelect=Low-pass  Filter_constant=0.01  advancedSettings=off  Ts=50e-6  cutOff_freq=32.1525
      settings: SourceProductBaseCode=MT
  Reversal : Step  Time=9
  Switch : Switch  Criteria=u2 > Threshold
  T_load : Step  Time=3  Before=0.05*acim.T_rated  After=0.3*acim.T_rated  SampleTime=Ts_simulink
  T_load1 : Step  Time=6  Before=0.3*acim.T_rated  After=-0.3*acim.T_rated  SampleTime=Ts_simulink
  Load_Trq : Outport  VectorParamsAs1DForOutWhenUnconnected=off
  wires:
  Switch/1 -> Data Type Conversion/1
  Data Type Conversion/1 -> IIR Filter/1
  IIR Filter/1 -> Load_Trq/1
  T_load1/1 -> Switch/1
  Reversal/1 -> Switch/2
  T_load/1 -> Switch/3

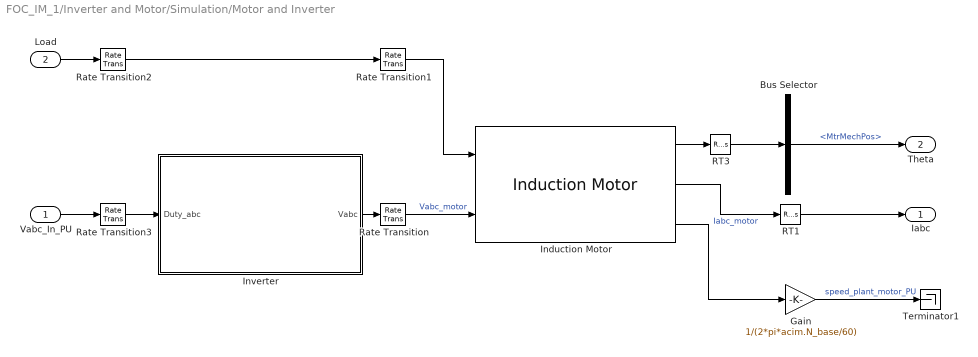
== system FOC_IM_1/Inverter and Motor/Simulation/Motor and Inverter ==
  Vabc_In_PU : Inport
  Load : Inport  Port=2
  Bus Selector : BusSelector  OutputSignals=MtrMechPos
  Gain : Gain  Gain=1/(2*pi*acim.N_base/60)
  Induction Motor : autolibim/Induction Motor  sim_type=Discrete  Ts=Ts_motor  port_config=Torque  P=acim.p  Zs=[acim.Rs, acim.Lls]  Zr=[acim.Rr, acim.Llr]  Lm=acim.Lm  mechanical=[acim.J, acim.B, 0]  theta_init=0  omega_init=0  RefBlkName='autolibim/Induction Motor'  aMode=5
      settings: SourceProductBaseCode=PW,DR,MT,UV,VE
  Inverter : Subsystem
  RT1 : RateTransition  Deterministic=off  OutPortSampleTime=Ts_simulink
  RT3 : RateTransition  Deterministic=off  OutPortSampleTime=Ts_simulink
  Rate Transition : RateTransition  Integrity=off  OutPortSampleTime=Ts_motor
  Rate Transition1 : RateTransition  Integrity=off  OutPortSampleTime=Ts_motor
  Rate Transition2 : RateTransition  Deterministic=off  OutPortSampleTime=Ts_inverter
  Rate Transition3 : RateTransition  Deterministic=off  OutPortSampleTime=Ts_inverter
  Terminator1 : Terminator
  Iabc : Outport
  Theta : Outport  Port=2
  wires:
  Rate Transition3/1 -> Inverter/1(Duty_abc)
  Rate Transition2/1 -> Rate Transition1/1
  Bus Selector/1 -> Theta/1  "<MtrMechPos>"
  RT3/1 -> Bus Selector/1
  RT1/1 -> Iabc/1
  Vabc_In_PU/1 -> Rate Transition3/1
  Inverter/1(Vabc) -> Rate Transition/1
  Rate Transition1/1 -> Induction Motor/1
  Induction Motor/2 -> RT1/1  "Iabc_motor"
  Rate Transition/1 -> Induction Motor/2  "Vabc_motor"
  Load/1 -> Rate Transition2/1
  Induction Motor/3 -> Gain/1
  Induction Motor/1 -> RT3/1
  Gain/1 -> Terminator1/1  "speed_plant_motor_PU"

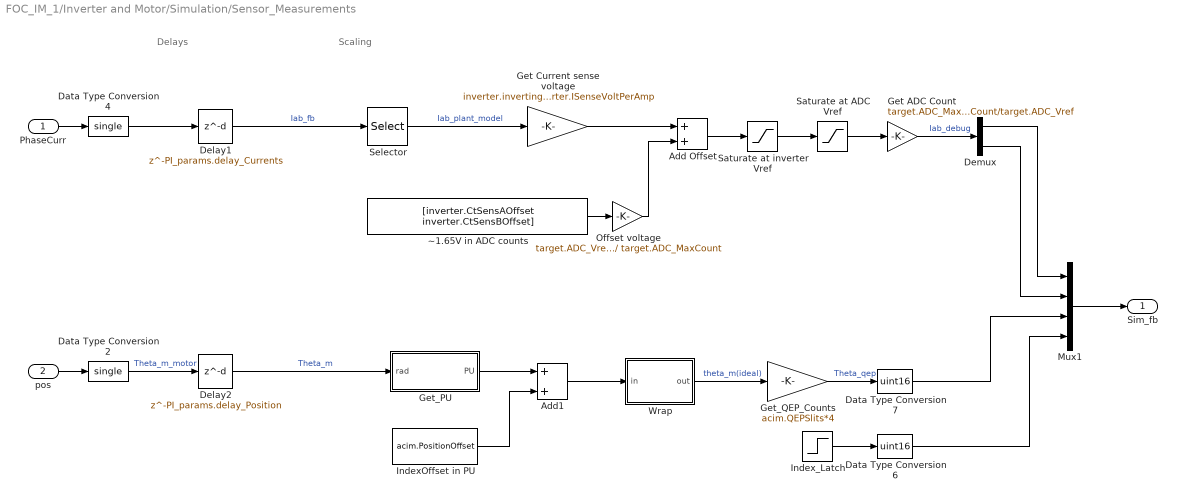
== system FOC_IM_1/Inverter and Motor/Simulation/Sensor_Measurements ==
  note: Scaling
  note: Delays
  PhaseCurr : Inport
  pos : Inport  Port=2
  Add Offset : Sum  RndMeth=Simplest
  Add1 : Sum  RndMeth=Simplest
  Data Type Conversion2 : DataTypeConversion  OutDataTypeStr=single  RndMeth=Simplest
  Data Type Conversion4 : DataTypeConversion  OutDataTypeStr=single  RndMeth=Simplest
  Data Type Conversion6 : DataTypeConversion  OutDataTypeStr=uint16  RndMeth=Simplest
  Data Type Conversion7 : DataTypeConversion  OutDataTypeStr=uint16  RndMeth=Simplest
  Delay1 : Delay  DelayLength=PI_params.delay_Currents
  Delay2 : Delay  DelayLength=PI_params.delay_Position
  Demux : Demux  Outputs=2
  Get ADC Count : Gain  Gain=target.ADC_MaxCount/target.ADC_Vref  OutMin=0  OutMax=target.ADC_MaxCount  OutDataTypeStr=uint16  RndMeth=Simplest
  Get Current sense voltage : Gain  Gain=inverter.invertingAmp * inverter.ISenseVoltPerAmp  RndMeth=Simplest  OutDataTypeStr=Inherit: Same as input
  "Get_PU " : Subsystem
  Get_QEP_Counts : Gain  Gain=acim.QEPSlits*4  OutDataTypeStr=uint16  RndMeth=Simplest
  IndexOffset in PU : Constant  Value=acim.PositionOffset  OutDataTypeStr=single  SampleTime=-1
  Index_Latch : Step  Time=Ts_motor  SampleTime=Ts_motor
  Mux1 : Mux
  Offset voltage : Gain  Gain=target.ADC_Vref / target.ADC_MaxCount  OutDataTypeStr=single  RndMeth=Simplest
  Saturate at ADC Vref : Saturate  UpperLimit=target.ADC_Vref  LowerLimit=0
  Saturate at inverter Vref : Saturate  UpperLimit=inverter.ISenseVref  LowerLimit=0
  Selector : Selector  InputPortWidth=3  IndexOptions=Index vector (dialog)  Indices=[1 2]  OutputSizes=1
  Wrap : Subsystem
  ~1.65V in ADC counts : Constant  Value=[inverter.CtSensAOffset inverter.CtSensBOffset]  OutDataTypeStr=uint16  SampleTime=-1
  Sim_fb : Outport  VectorParamsAs1DForOutWhenUnconnected=off
  wires:
  Delay1/1 -> Selector/1  "Iab_fb"
  Data Type Conversion4/1 -> Delay1/1
  Selector/1 -> Get Current sense voltage/1  "Iab_plant_model"
  PhaseCurr/1 -> Data Type Conversion4/1
  Demux/1 -> Mux1/1
  Mux1/1 -> Sim_fb/1
  Demux/2 -> Mux1/2
  Data Type Conversion2/1 -> Delay2/1  "Theta_m_motor"
  Add1/1 -> Wrap/1(in)
  Delay2/1 -> "Get_PU "/1(rad)  "Theta_m"
  Wrap/1(out) -> Get_QEP_Counts/1  "theta_m(ideal)"
  Get_QEP_Counts/1 -> Data Type Conversion7/1  "Theta_qep"
  IndexOffset in PU/1 -> Add1/2
  Data Type Conversion7/1 -> Mux1/3
  Data Type Conversion6/1 -> Mux1/4
  Index_Latch/1 -> Data Type Conversion6/1
  pos/1 -> Data Type Conversion2/1
  Get ADC Count/1 -> Demux/1  "Iab_debug"
  "Get_PU "/1(PU) -> Add1/1
  Get Current sense voltage/1 -> Add Offset/1
  Add Offset/1 -> Saturate at inverter Vref/1
  Saturate at ADC Vref/1 -> Get ADC Count/1
  Saturate at inverter Vref/1 -> Saturate at ADC Vref/1
  Offset voltage/1 -> Add Offset/2
  ~1.65V in ADC counts/1 -> Offset voltage/1

== system FOC_IM_1/Serial Receive/Data_Conditioning_Rx/Data_Type_Float ==
  In1 : Inport
  Data Type Conversion2 : DataTypeConversion  OutDataTypeStr=uint16  RndMeth=Simplest
  Demux : Demux  Outputs=2
  Out1 : Outport
  Out2 : Outport  Port=2
  wires:
  In1/1 -> Demux/1
  Demux/1 -> Out1/1
  Data Type Conversion2/1 -> Out2/1
  Demux/2 -> Data Type Conversion2/1

== system FOC_IM_1/Serial Receive/Simulation/Data_Conditioning_Tx ==
  In1 : Inport
  In2 : Inport  Port=2
  Data_Type_Float : Subsystem  VariantControl=isequal(dataType, 'single')
  Data : Outport

== system FOC_IM_1/Serial Receive/Simulation/Parse ==
  Enable_PWM : Inport
  Enable_FWC : Inport  Port=2
  Debug_signals : Inport  Port=3
  Bitwise Operator : simulink/Logic and Bit Operations/Bitwise Operator  logicop=AND  UseBitMask=on  BitMask=hex2dec('0001')  BitMaskRealWorld=Stored Integer
  Bitwise Operator1 : simulink/Logic and Bit Operations/Bitwise Operator  logicop=AND  UseBitMask=on  BitMask=hex2dec('00F0')  BitMaskRealWorld=Stored Integer
  Bitwise Operator2 : simulink/Logic and Bit Operations/Bitwise Operator  logicop=AND  UseBitMask=on  BitMask=hex2dec('0002')  BitMaskRealWorld=Stored Integer
  Shift Arithmetic : ArithShift  BitShiftNumber=-1
  Shift Arithmetic1 : ArithShift  BitShiftNumber=-4
  Sum : Sum  Inputs=|+++
  Data : Outport
  wires:
  Bitwise Operator/1 -> Sum/1
  Debug_signals/1 -> Shift Arithmetic1/1
  Sum/1 -> Data/1
  Shift Arithmetic1/1 -> Bitwise Operator1/1
  Enable_PWM/1 -> Bitwise Operator/1
  Shift Arithmetic/1 -> Bitwise Operator2/1
  Bitwise Operator1/1 -> Sum/3
  Enable_FWC/1 -> Shift Arithmetic/1
  Bitwise Operator2/1 -> Sum/2

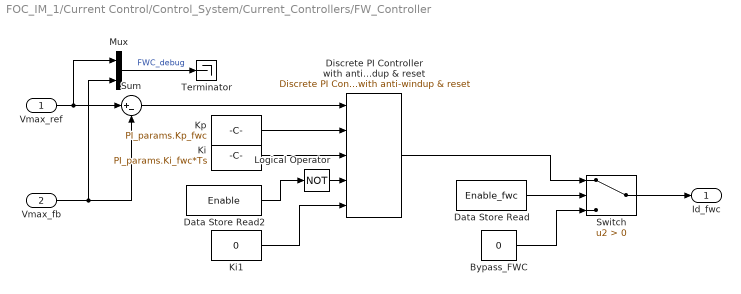
== system FOC_IM_1/Current Control/Control_System/Current_Controllers/FW_Controller ==
  Vmax_ref : Inport
  Vmax_fb : Inport  Port=2
  Bypass_FWC : Constant  Value=0  OutDataTypeStr=Inherit: Inherit via back propagation  SampleTime=-1
  Data Store Read : DataStoreRead  DataStoreName=Enable_fwc  IndexOptions=Index vector (dialog)  Indices=1  OutputSizes=1
  Data Store Read2 : DataStoreRead  DataStoreName=Enable  IndexOptions=Index vector (dialog)  Indices=1  OutputSizes=1
  Discrete PI Controller with anti-windup & reset : mcbcontrolslib/Discrete PI Controller  with anti-windup & reset  UpperSaturationLimit=0  LowerSaturationLimit=-0.5
      settings: SourceProductBaseCode=MT
  Ki : Constant  Value=PI_params.Ki_fwc*Ts  OutDataTypeStr=dataType  SampleTime=-1
  Ki1 : Constant  Value=0  OutDataTypeStr=dataType  SampleTime=-1
  Kp : Constant  Value=PI_params.Kp_fwc  OutDataTypeStr=dataType  SampleTime=-1
  Logical Operator : Logic  Operator=NOT  IconShape=distinctive  AllPortsSameDT=off  OutDataTypeStr=boolean
  Mux : Mux  Inputs=2
  Sum : Sum  Inputs=|+-  OutDataTypeStr=Inherit: Same as first input
  Switch : Switch  Criteria=u2 > Threshold
  Terminator : Terminator
  Id_fwc : Outport  VectorParamsAs1DForOutWhenUnconnected=off
  wires:
  Vmax_fb/1 -> Sum/2, Mux/2
  Kp/1 -> Discrete PI Controller with anti-windup & reset/2
  Ki/1 -> Discrete PI Controller with anti-windup & reset/3
  Ki1/1 -> Discrete PI Controller with anti-windup & reset/5
  Mux/1 -> Terminator/1  "FWC_debug"
  Bypass_FWC/1 -> Switch/3
  Switch/1 -> Id_fwc/1
  Data Store Read2/1 -> Logical Operator/1
  Logical Operator/1 -> Discrete PI Controller with anti-windup & reset/4
  Sum/1 -> Discrete PI Controller with anti-windup & reset/1
  Vmax_ref/1 -> Mux/1, Sum/1
  Data Store Read/1 -> Switch/2
  Discrete PI Controller with anti-windup & reset/1 -> Switch/1

== system FOC_IM_1/Current Control/Control_System/Current_Controllers/PI_Controller_Id ==
  I_ref : Inport
  I_fb : Inport  Port=2
  Data Store Read1 : DataStoreRead  DataStoreName=Enable  IndexOptions=Index vector (dialog)  Indices=1  OutputSizes=1
  Discrete PI Controller with anti-windup & reset : mcbcontrolslib/Discrete PI Controller  with anti-windup & reset  UpperSaturationLimit=1  LowerSaturationLimit=-1
      settings: SourceProductBaseCode=MT
  Initial_Condition : Constant  Value=0  OutDataTypeStr=dataType  SampleTime=-1
  Ki : Constant  Value=PI_params.Ki_id*Ts  OutDataTypeStr=dataType  SampleTime=-1
  Kp : Constant  Value=PI_params.Kp_id  OutDataTypeStr=dataType  SampleTime=-1
  Logical Operator : Logic  Operator=NOT  IconShape=distinctive  AllPortsSameDT=off  OutDataTypeStr=boolean
  Sum : Sum  Inputs=|+-  OutDataTypeStr=Inherit: Same as first input
  Vd_ref : Outport  VectorParamsAs1DForOutWhenUnconnected=off
  wires:
  I_fb/1 -> Sum/2
  I_ref/1 -> Sum/1
  Ki/1 -> Discrete PI Controller with anti-windup & reset/3
  Logical Operator/1 -> Discrete PI Controller with anti-windup & reset/4
  Sum/1 -> Discrete PI Controller with anti-windup & reset/1
  Kp/1 -> Discrete PI Controller with anti-windup & reset/2
  Discrete PI Controller with anti-windup & reset/1 -> Vd_ref/1
  Data Store Read1/1 -> Logical Operator/1
  Initial_Condition/1 -> Discrete PI Controller with anti-windup & reset/5

== system FOC_IM_1/Current Control/Control_System/Current_Controllers/PI_Controller_Iq ==
  I_ref : Inport
  I_fb : Inport  Port=2
  Data Store Read1 : DataStoreRead  DataStoreName=Enable  IndexOptions=Index vector (dialog)  Indices=1  OutputSizes=1
  Discrete PI Controller with anti-windup & reset : mcbcontrolslib/Discrete PI Controller  with anti-windup & reset  UpperSaturationLimit=1  LowerSaturationLimit=-1
      settings: SourceProductBaseCode=MT
  Initial_Condition : Constant  Value=0  OutDataTypeStr=dataType  SampleTime=-1
  Ki : Constant  Value=PI_params.Ki_i*Ts  OutDataTypeStr=dataType  SampleTime=-1
  Kp : Constant  Value=PI_params.Kp_i  OutDataTypeStr=dataType  SampleTime=-1
  Logical Operator : Logic  Operator=NOT  IconShape=distinctive  AllPortsSameDT=off  OutDataTypeStr=boolean
  Sum : Sum  Inputs=|+-  OutDataTypeStr=Inherit: Same as first input
  Vq_ref : Outport  VectorParamsAs1DForOutWhenUnconnected=off
  wires:
  I_fb/1 -> Sum/2
  I_ref/1 -> Sum/1
  Ki/1 -> Discrete PI Controller with anti-windup & reset/3
  Logical Operator/1 -> Discrete PI Controller with anti-windup & reset/4
  Sum/1 -> Discrete PI Controller with anti-windup & reset/1
  Kp/1 -> Discrete PI Controller with anti-windup & reset/2
  Discrete PI Controller with anti-windup & reset/1 -> Vq_ref/1
  Data Store Read1/1 -> Logical Operator/1
  Initial_Condition/1 -> Discrete PI Controller with anti-windup & reset/5

== system FOC_IM_1/Current Control/HW_Inputs/Sensor Driver Blocks (codegen)/Optional_Read_SPI ==
  Data Type Conversion1 : DataTypeConversion  OutDataTypeStr=uint32  ConvertRealWorld=Stored Integer (SI)  RndMeth=Simplest
  Mux3 : Mux  Inputs=2
  Read_ADC_Gain : Constant  Priority=2000  Value=0xD000  OutDataTypeStr=uint16  SampleTime=-1
  Read_PWM_mode : Constant  Priority=2000  Value=0xB800  OutDataTypeStr=uint16  SampleTime=-1
  SPI Master Transfer2 : c280xlib/SPI Master Transfer  SPISelect=SPI_A  ClockPolarity=Rising_edge  ClockPhase=No_delay  SPIModule=uint32(0)  Mode=Master  BusSpeed=uint32(1000000)  FirstBitToTransfer=Most significant bit (MSB)  ClockMode=0  BlockFunction=Transfer  EnableRegisterAddress=off  RegisterAddress=0  OutputDataType=int8  OutputDataLength=1  DataBits=16  UseCustomSSPin=Provided by the SPI peripheral  ActiveLowSSPin=Active low  Pin=61
      settings: SourceProductBaseCode=TIC2000
  SPI Master Transfer5 : c280xlib/SPI Master Transfer  SPISelect=SPI_A  ClockPolarity=Rising_edge  ClockPhase=No_delay  SPIModule=uint32(0)  Mode=Master  BusSpeed=uint32(1000000)  FirstBitToTransfer=Most significant bit (MSB)  ClockMode=0  BlockFunction=Transfer  EnableRegisterAddress=off  RegisterAddress=0  OutputDataType=int8  OutputDataLength=1  DataBits=16  UseCustomSSPin=Provided by the SPI peripheral  ActiveLowSSPin=Active low  Pin=61
      settings: SourceProductBaseCode=TIC2000
  Read_SPI : Outport
  wires:
  Read_PWM_mode/1 -> SPI Master Transfer5/1
  Read_ADC_Gain/1 -> SPI Master Transfer2/1
  SPI Master Transfer2/1 -> Mux3/2
  SPI Master Transfer5/1 -> Mux3/1
  Mux3/1 -> Data Type Conversion1/1
  Data Type Conversion1/1 -> Read_SPI/1

== system FOC_IM_1/Current Control/Input Scaling/Calculate Phase Currents/Data_Type ==
  In1 : Inport
  Data_Type_Float : Subsystem  VariantControl=isequal(dataType,'single')
  Out1 : Outport

== system FOC_IM_1/Inverter and Motor/Simulation/Motor and Inverter/Inverter ==
  Duty_abc : Inport
  Average-Value Inverter : mcbplantlib/Average-Value Inverter
  Constant2 : Constant  Value=inverter.V_dc  OutDataTypeStr=single  SampleTime=-1
  Data Type Conversion1 : DataTypeConversion  OutDataTypeStr=single  RndMeth=Simplest
  Vabc : Outport  VectorParamsAs1DForOutWhenUnconnected=off
  wires:
  Constant2/1 -> Average-Value Inverter/2
  Data Type Conversion1/1 -> Average-Value Inverter/1
  Duty_abc/1 -> Data Type Conversion1/1
  Average-Value Inverter/1 -> Vabc/1  "Vabc"

== system FOC_IM_1/Inverter and Motor/Simulation/Sensor_Measurements/Get_PU  ==
  rad : Inport
  Constant2 : Constant  Value=2*pi  OutDataTypeStr=single  SampleTime=-1
  Get_PU : Gain  Gain=1/(2*pi)  RndMeth=Simplest  OutDataTypeStr=Inherit: Same as input
  Mod : Math  Operator=mod  SaturateOnIntegerOverflow=on
  PU : Outport  VectorParamsAs1DForOutWhenUnconnected=off
  wires:
  rad/1 -> Mod/1
  Constant2/1 -> Mod/2
  Mod/1 -> Get_PU/1
  Get_PU/1 -> PU/1

== system FOC_IM_1/Inverter and Motor/Simulation/Sensor_Measurements/Wrap ==
  in : Inport
  Constant2 : Constant  OutDataTypeStr=single  SampleTime=-1
  Mod : Math  Operator=mod  SaturateOnIntegerOverflow=on
  out : Outport  VectorParamsAs1DForOutWhenUnconnected=off
  wires:
  in/1 -> Mod/1
  Constant2/1 -> Mod/2
  Mod/1 -> out/1

== system FOC_IM_1/Serial Receive/Simulation/Data_Conditioning_Tx/Data_Type_Float ==
  In1 : Inport
  In2 : Inport  Port=2
  Data Type Conversion2 : DataTypeConversion  OutDataTypeStr=single  RndMeth=Simplest
  Mux : Mux  Inputs=2
  Data : Outport
  wires:
  In1/1 -> Mux/1
  Mux/1 -> Data/1
  In2/1 -> Data Type Conversion2/1
  Data Type Conversion2/1 -> Mux/2

== system FOC_IM_1/Current Control/Input Scaling/Calculate Phase Currents/Data_Type/Data_Type_Float ==
  In1 : Inport
  Get ADC Voltage : Gain  Gain=target.ADC_Vref /target.ADC_MaxCount  OutDataTypeStr=dataType  RndMeth=Simplest
  Get Currents : Gain  Gain=1/inverter.ISenseVoltPerAmp  RndMeth=Simplest  OutDataTypeStr=Inherit: Same as input
  PU_Conversion : Gain  Gain=1/PU_System.I_base  RndMeth=Simplest  OutDataTypeStr=Inherit: Same as input
  Out1 : Outport
  wires:
  Get ADC Voltage/1 -> Get Currents/1
  Get Currents/1 -> PU_Conversion/1
  In1/1 -> Get ADC Voltage/1
  PU_Conversion/1 -> Out1/1

== matlab function FOC_IM_1/Speed Control/MATLAB Function ==
  data: E input; T_ref output; I input
function T_ref = fcn(E,I)
NE=0; NI=0; PI=0; PE=0; NN=0; NP=0; PN=0; PP=0;
% Fuzzy Logic
% PI Controller
% 4 Fuzzy Rules
% BE Error Break Point
% BI Integral Break Point
% Signal Break Points
% BQ1 BQ2
% Error E Integral D Control Q
% IF E IS N && I IS N THEN Q IS NN
% IF E IS N && I IS P THEN Q IS NP
% IF E IS P && I IS N THEN Q IS PN
% IF E IS P && I IS P THEN Q IS PP
% Data
BE=15; BI=0.5;
BQ1=10; BQ2=40;
GQ1=BQ1; GQ2=BQ2-BQ1;
HQ1=BQ1/2;HQ2=BQ1+(BQ2-BQ1)/2;
% Calculations
% Input Membership Values
if(E<-BE) NE=1.0; PE=0.0; end;
if(E>+BE) NE=0.0; PE=1.0; end;
if(E>=-BE && E<=+BE)
NE=1-(E+BE)/(2*BE);
PE=(E+BE)/(2*BE);
end;
if(I<-BI) NI=1.0; PI=0.0; end;
if(I>+BI) NI=0.0; PI=1.0; end;
if(I>=-BI && I<=+BI)
NI=1-(I+BI)/(2*BI);
PI=(I+BI)/(2*BI);
end;
% Output Membership Values
if(NE<NI) NN=NE; end;
if(NE>=NI) NN=NI; end;
if(NE<PI) NP=NE; end;
if(NE>=PI) NP=PI; end;
if(PE<NI) PN=PE; end;
if(PE>=NI) PN=NI; end;
if(PE<PI) PP=PE; end;
if(PE>=PI) PP=PI; end;
% Defuzzification
T_ref=(-NN*GQ2*HQ2-NP*GQ1*HQ1+PN*GQ1*HQ1+PP*GQ2*HQ2)/(NN*GQ2+NP*GQ1+PN*GQ1+PP*GQ2)
